simulink model "ch_11_design_algo_examples"  (R2022b)
settings: Solver=VariableStepAuto  StartTime=0.0  StopTime=5  RelTol=1e-3
settings Model: Creator=Mahadevu Sudheer  LastModifiedBy=Mahadevu Sudheer

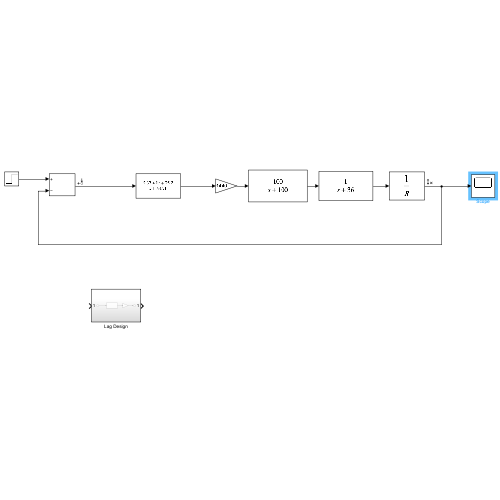
[thumbnail: Simulink's stored preview of the top-level diagram]
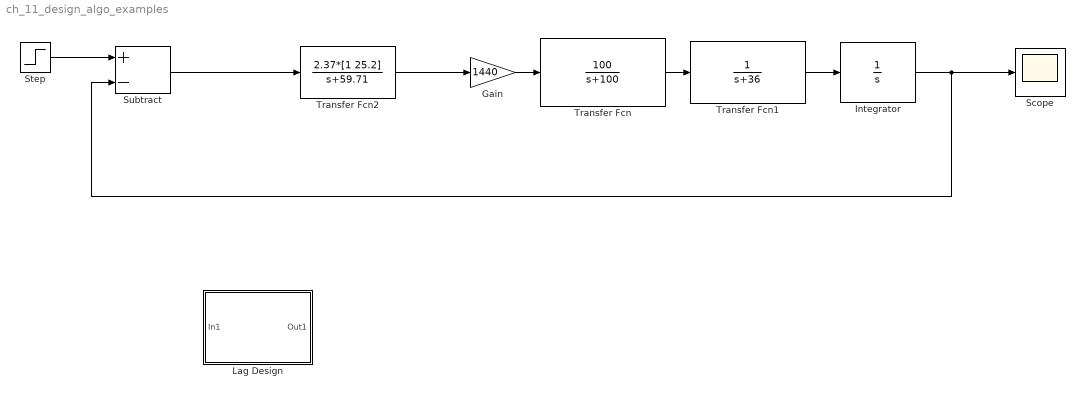
== system ch_11_design_algo_examples ==
  Gain : Gain  Gain=1440
  Integrator : Integrator
  Lag Design : Subsystem
  Scope : Scope
  Step : Step  Time=0  SampleTime=0
  Subtract : Sum  Inputs=+-
  Transfer Fcn : TransferFcn  Numerator=[100]  Denominator=[1 100]
  Transfer Fcn1 : TransferFcn  Denominator=[1 36]
  Transfer Fcn2 : TransferFcn  Numerator=2.37*[1 25.2]  Denominator=[1 59.71]
  wires:
  Transfer Fcn/1 -> Transfer Fcn1/1
  Transfer Fcn1/1 -> Integrator/1
  Integrator/1 -> Subtract/2, Scope/1
  Step/1 -> Subtract/1
  Gain/1 -> Transfer Fcn/1
  Subtract/1 -> Transfer Fcn2/1
  Transfer Fcn2/1 -> Gain/1

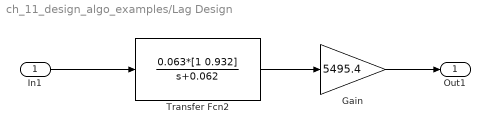
== system ch_11_design_algo_examples/Lag Design ==
  In1 : Inport
  Gain : Gain  Gain=5495.4
  Transfer Fcn2 : TransferFcn  Numerator=0.063*[1 0.932]  Denominator=[1 0.062]
  Out1 : Outport
  wires:
  Transfer Fcn2/1 -> Gain/1
  Gain/1 -> Out1/1
  In1/1 -> Transfer Fcn2/1
